simulink subsystem "RW_DYNAMICS"  (R2025b)
settings: Solver=VariableStepAuto  StartTime=0.0  StopTime=10.0  RelTol=1e-3
model mask{Js=0, Jw=0, x0=0}
  mask prompts: Js "Satellite inertia [kgm2]"; Jw "RW inertia [kgm2]"; x0 "Initial state vector [rad, rad/s, rad/s]"
values from neighbouring files (symbols this model uses):
  x0 = [initSatPhi; initSatAngVel; initWheelAngVel] .* (pi / 180)    [input_script.m]
settings Model: Creator=antoniohernandez-rodiciomateos  LastModifiedBy=antoniohernandez-rodiciomateos

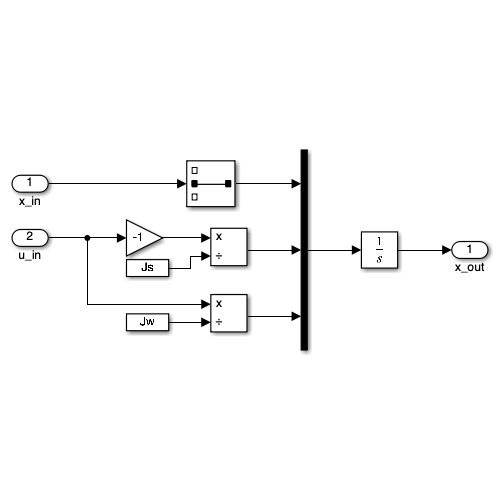
[thumbnail: Simulink's stored preview of the top-level diagram]
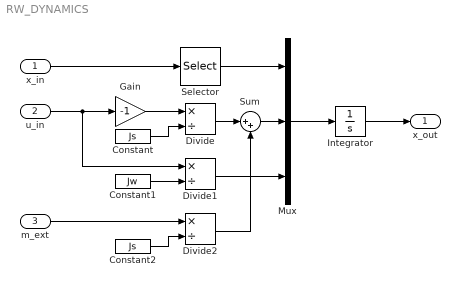
== system RW_DYNAMICS ==
  x_in : Inport
  u_in : Inport  Port=2
  m_ext : Inport  Port=3
  Constant : Constant  Value=Js
  Constant1 : Constant  Value=Jw
  Constant2 : Constant  Value=Js
  Divide : Product  Inputs=*/
  Divide1 : Product  Inputs=*/
  Divide2 : Product  Inputs=*/
  Gain : Gain  Gain=-1
  Integrator : Integrator  InitialCondition=x0
  Mux : Mux  Inputs=3
  Selector : Selector  InputPortWidth=3  IndexOptions=Index vector (dialog)  Indices=[2]  OutputSizes=1
  Sum : Sum  Inputs=|++
  x_out : Outport
  wires:
  x_in/1 -> Selector/1
  Selector/1 -> Mux/1
  u_in/1 -> Divide1/1, Gain/1
  Gain/1 -> Divide/1
  Constant/1 -> Divide/2
  Constant1/1 -> Divide1/2
  Divide1/1 -> Mux/3
  Mux/1 -> Integrator/1
  Integrator/1 -> x_out/1
  m_ext/1 -> Divide2/1
  Constant2/1 -> Divide2/2
  Divide/1 -> Sum/1
  Sum/1 -> Mux/2
  Divide2/1 -> Sum/2
